simulink model "program_nova_torque_vectoring_001_2015b"  (R2016a)
settings: Solver=FixedStepAuto  StartTime=0.0  StopTime=10.0  RelTol=1e-3
PreLoadFcn:
  | dataCar
  | load_vars
  | readFuzzyFile
  | structAero
  | structEstimPar
  | structSensors
  | structSettings
PostLoadFcn:
  | , if any(exist('dsrtsu_mdlpostloadfcn', 'file') == [2, 3, 6]), try dsrtsu_mdlpostloadfcn('Execute', bdroot); catch fprintf('Error in PostLoadFcn (dsrtsu_mdlpostloadfcn) for model "%s":\n %s\n', bdroot, lasterr); end, end,
InitFcn:
  | dataCar
  | load_vars
  | readFuzzyFile
  | structAero
  | structEstimPar
  | structSensors
  | structSettings
StartFcn:
  | dataCar
  | load_vars
  | readFuzzyFile
  | structAero
  | structEstimPar
  | structSensors
  | structSettings
values from neighbouring files (symbols this model uses):
  Throttle2_offset = 500    [load_vars.m]
  Throttle_limits = [0.15, 0.90, 0.16, 0.92]    [load_vars.m]
libraries: rtican x42, hdlsllib x32, simulink x3, fuzblock x1
(part 6 of 11)

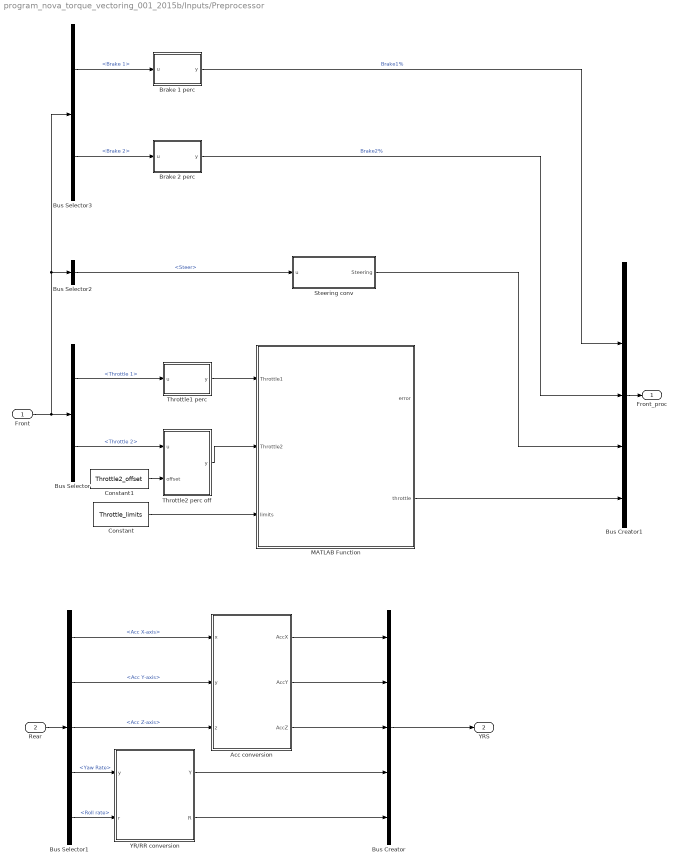
== system program_nova_torque_vectoring_001_2015b/Inputs/Preprocessor ==
  Front : Inport
  Rear : Inport  Port=2
  Acc conversion : MATLAB Function  TreatAsAtomicUnit=on
  "Brake 1 perc " : MATLAB Function  TreatAsAtomicUnit=on
  "Brake 2 perc " : MATLAB Function  TreatAsAtomicUnit=on
  Bus Creator : BusCreator  Inputs=5
  Bus Creator1 : BusCreator  Inputs=5
  Bus Selector : BusSelector  OutputSignals=Throttle 1,Throttle 2
  Bus Selector1 : BusSelector  OutputSignals=Acc X-axis,Acc Y-axis,Acc Z-axis,Yaw Rate,Roll rate
  Bus Selector2 : BusSelector  OutputSignals=Steer
  Bus Selector3 : BusSelector  OutputSignals=Brake 1,Brake 2
  Constant : Constant  Value=Throttle_limits
  Constant1 : Constant  Value=Throttle2_offset
  MATLAB Function : MATLAB Function  TreatAsAtomicUnit=on
  Steering conv : MATLAB Function  TreatAsAtomicUnit=on
  Throttle1 perc : MATLAB Function  TreatAsAtomicUnit=on
  Throttle2 perc off : MATLAB Function  TreatAsAtomicUnit=on
  YR/RR conversion : MATLAB Function  TreatAsAtomicUnit=on
  Front_proc : Outport
  YRS : Outport  Port=2
  wires:
  Front/1 -> Bus Selector3/1, Bus Selector2/1, Bus Selector/1
  Constant/1 -> MATLAB Function/3(limits)
  Bus Selector/2 -> Throttle2 perc off/1(u)  "<Throttle 2>"
  Throttle2 perc off/1(y) -> MATLAB Function/2(Throttle2)
  Bus Selector/1 -> Throttle1 perc/1(u)  "<Throttle 1>"
  Throttle1 perc/1(y) -> MATLAB Function/1(Throttle1)
  Constant1/1 -> Throttle2 perc off/2(offset)
  MATLAB Function/2(throttle) -> Bus Creator1/5
  Rear/1 -> Bus Selector1/1
  Bus Selector1/1 -> Acc conversion/1(x)  "<Acc X-axis>"
  Bus Selector1/2 -> Acc conversion/2(y)  "<Acc Y-axis>"
  Bus Selector1/3 -> Acc conversion/3(z)  "<Acc Z-axis>"
  Bus Selector1/4 -> YR/RR conversion/1(y)  "<Yaw Rate>"
  Bus Selector1/5 -> YR/RR conversion/2(r)  "<Roll rate>"
  Acc conversion/3(AccZ) -> Bus Creator/3
  Acc conversion/2(AccY) -> Bus Creator/2
  Acc conversion/1(AccX) -> Bus Creator/1
  YR/RR conversion/1(Y) -> Bus Creator/4
  YR/RR conversion/2(R) -> Bus Creator/5
  Bus Creator/1 -> YRS/1
  Bus Selector2/1 -> Steering conv/1(u)  "<Steer>"
  Steering conv/1(Steering) -> Bus Creator1/4
  Bus Selector3/1 -> "Brake 1 perc "/1(u)  "<Brake 1>"
  Bus Selector3/2 -> "Brake 2 perc "/1(u)  "<Brake 2>"
  "Brake 2 perc "/1(y) -> Bus Creator1/3  "Brake2%"
  "Brake 1 perc "/1(y) -> Bus Creator1/2  "Brake1%"
  Bus Creator1/1 -> Front_proc/1
